simulink model "RemoteMicrogrid"  (R2025a)
settings: Solver=FixedStepAuto  StartTime=0.0  StopTime=8  FixedStep=Ts  MaxStep=1e-3  RelTol=1e-3
PreLoadFcn:
  | RemoteMicrogridInputData
undefined symbols (not defined in the file): BESS, ControlRoom, DiscIntNeverNeededParam, Grid, Load, Machine, Microgrid, MicrogridStatus, PV, relay1, T_on, Ts
libraries: ee_lib x53, fl_lib x39, eeGeneralControl x30, simulink x30, nesl_utility x26, nesl_utility_internal x19, slpidlib x7, eeTransforms x5, eeRmsMeasurement x4, eeTotalHarmonicDistorsion x4, batteryecm_lib x2, simulink_extras x2
(part 4 of 6)

== system RemoteMicrogrid/Diesel Substation, BESS, & Microgrid Controller/Diesel Generator/AVR and Exciter ==
  Constant{3,5..9} (6 alike) : Constant  Value=0
  Constant4 : Constant  Value=1.05
  "E_FD Simulink-PS " : nesl_utility/Simulink-PS Converter  PhysicalDomain=network_engine_domain  SubClassName=ps_input  LeftPortType=input  RightPortType=output  PseudoPeriodic=off  Frequencies=[]  NoiseDistribution=none  NoiseParameters=[]  Unit=1  AffineConversion=off  FilteringAndDerivatives=provide  SimscapeFilterOrder=1  InputFilterTimeConstant=.001  UdotUserProvided=0
  I_FD PS-Simulink : nesl_utility/PS-Simulink Converter  PhysicalDomain=network_engine_domain  SubClassName=ps_output  LeftPortType=input  RightPortType=output  PseudoPeriodic=off  Frequencies=[]  VectorFormat=1-D array  Unit=1  AffineConversion=off
  SM DC2C : eeSmDC2C/SM DC2C  E_FD0=2.5  Ts=Ts  R_C=0  X_C=0  T_R=0  K_A=300  T_A=0.06  T_B=0  T_C=0  K_F=0.058  T_F=0.62  V_Rmax=4.5  V_Rmin=-4.5  oelInputLocation=Unused  uelInputLocation=Unused  sclInputLocation=Unused  K_E=1  T_E=1.33  E_FDmin=-99  E_1=3.05  S_E_E1=0.279  E_2=2.29  S_E_E2=0.117
  Synchronous Machine Field Circuit (pu) : ee_lib/Electromechanical/Synchronous/Synchronous Machine Field Circuit  unit_option=ee.enum.unit.pu  SRated=Grid.DieselRatedPower V*A  FRated=Grid.Frequency Hz  fieldCircuitParameterization_option=ee.enum.sm.fieldparameterization.current  baseEfd=200 V  baseIfd=1300 A  parameterization_option=2  Ladu=1.66  Rfd=0.0006  Xl=0.05  Xd=1.72  Xdd=0.13  Xddd=0.09  d_option=ee.enum.circuit.open  Td0d=0.75 s  Tdd=0.03 s  Td0dd=0.003 s  Tddd=0.008 s
      settings: InternalSimscapePortConfiguration="{\"Bottom\":[],\"Left\":[{\"id\":\"Efd_pu\",\"label\":\"Efd_pu\",\"type\":\"input\"},{\"id\":\"Ifd_pu\",\"label\":\"Ifd_pu\",\"type\":\"output\"}],\"Right\":[{\"id\":\"fd_p\",\"label\":\"fd+\",\"type\":\"foundation.electrical.electrical\"},{\"id\":\"fd_n\",\"label\":\"fd-\",\"type\":\"foundation.electrical.electrical\"}],\"Top\":[]}"
  Terminal Current Measurement : ee_lib/Electromechanical/Synchronous/Synchronous Machine Measurement  output_idx=15
      settings: InternalSimscapePortConfiguration="{\"Bottom\":[],\"Left\":[{\"id\":\"pu_input\",\"label\":\"pu\",\"type\":\"input\"}],\"Right\":[{\"id\":\"pu_output\",\"label\":\"o\",\"type\":\"output\"}],\"Top\":[]}"
  Terminal Current PS-Simulink : nesl_utility/PS-Simulink Converter  PhysicalDomain=network_engine_domain  SubClassName=ps_output  LeftPortType=input  RightPortType=output  PseudoPeriodic=off  Frequencies=[]  VectorFormat=1-D array  Unit=1  AffineConversion=off
  Terminal Voltage Measurement : ee_lib/Electromechanical/Synchronous/Synchronous Machine Measurement  output_idx=14
      settings: InternalSimscapePortConfiguration="{\"Bottom\":[],\"Left\":[{\"id\":\"pu_input\",\"label\":\"pu\",\"type\":\"input\"}],\"Right\":[{\"id\":\"pu_output\",\"label\":\"o\",\"type\":\"output\"}],\"Top\":[]}"
  Terminal Voltage PS-Simulink : nesl_utility/PS-Simulink Converter  PhysicalDomain=network_engine_domain  SubClassName=ps_output  LeftPortType=input  RightPortType=output  PseudoPeriodic=off  Frequencies=[]  VectorFormat=1-D array  Unit=1  AffineConversion=off
  Terminator : Terminator
  pu : PMIOPort  Side=Left
  fd+ : PMIOPort  Port=2  Side=Right
  fd- : PMIOPort  Port=3  Side=Right
  wires:
  Terminal Current PS-Simulink/1 -> SM DC2C/4
  SM DC2C/1 -> "E_FD Simulink-PS "/1
  Constant9/1 -> SM DC2C/9
  Constant8/1 -> SM DC2C/8
  Constant7/1 -> SM DC2C/7
  Constant6/1 -> SM DC2C/6
  Constant5/1 -> SM DC2C/5
  Constant3/1 -> SM DC2C/2
  I_FD PS-Simulink/1 -> Terminator/1
  Constant4/1 -> SM DC2C/1
  Terminal Voltage PS-Simulink/1 -> SM DC2C/3
  connections:
  Terminal Current Measurement/RConn1 -- Terminal Current PS-Simulink/LConn1
  Terminal Voltage Measurement/RConn1 -- Terminal Voltage PS-Simulink/LConn1
  pu/RConn1 -- Terminal Current Measurement/LConn1 -- Terminal Voltage Measurement/LConn1
  Synchronous Machine Field Circuit (pu)/RConn1 -- fd+/RConn1
  fd-/RConn1 -- Synchronous Machine Field Circuit (pu)/RConn2
  I_FD PS-Simulink/LConn1 -- Synchronous Machine Field Circuit (pu)/LConn2
  "E_FD Simulink-PS "/RConn1 -- Synchronous Machine Field Circuit (pu)/LConn1

== system RemoteMicrogrid/Diesel Substation, BESS, & Microgrid Controller/Diesel Generator/Governor and Prime Mover  ==
  Load : Inport
  Governor : Subsystem
  Ideal Torque Source : fl_lib/Mechanical/Mechanical Sources/Ideal Torque Source
  Mechanical Rotational Reference : fl_lib/Mechanical/Rotational Elements/Mechanical Rotational Reference
  Non-reheat turbine : Subsystem
  PS-Simulink Converter : nesl_utility/PS-Simulink Converter  PhysicalDomain=network_engine_domain  SubClassName=ps_output  LeftPortType=input  RightPortType=output  PseudoPeriodic=off  Frequencies=[]  VectorFormat=1-D array  Unit=1  AffineConversion=off
  Rotor Velocity Measurement : ee_lib/Electromechanical/Synchronous/Synchronous Machine Measurement  output_idx=4
      settings: InternalSimscapePortConfiguration="{\"Bottom\":[],\"Left\":[{\"id\":\"pu_input\",\"label\":\"pu\",\"type\":\"input\"}],\"Right\":[{\"id\":\"pu_output\",\"label\":\"o\",\"type\":\"output\"}],\"Top\":[]}"
  Simulink-PS Converter : nesl_utility/Simulink-PS Converter  PhysicalDomain=network_engine_domain  SubClassName=ps_input  LeftPortType=input  RightPortType=output  PseudoPeriodic=off  Frequencies=[]  NoiseDistribution=none  NoiseParameters=[]  Unit=1  AffineConversion=off  FilteringAndDerivatives=zero  SimscapeFilterOrder=1  InputFilterTimeConstant=0.001  UdotUserProvided=1
  scale by base_torque : Gain  Gain=base_torque
  R : PMIOPort  Side=Right
  C : PMIOPort  Port=2  Side=Right
  pu : PMIOPort  Port=3  Side=Left
  wires:
  PS-Simulink Converter/1 -> Governor/1(pu_velocity)
  Governor/1(delta_y) -> Non-reheat turbine/1(delta_y)
  Non-reheat turbine/1(torque) -> scale by base_torque/1
  scale by base_torque/1 -> Simulink-PS Converter/1
  Load/1 -> Governor/2(Load Reference)
  connections:
  C/RConn1 -- Ideal Torque Source/RConn2 -- Mechanical Rotational Reference/LConn1
  Ideal Torque Source/LConn1 -- R/RConn1
  pu/RConn1 -- Rotor Velocity Measurement/LConn1
  PS-Simulink Converter/LConn1 -- Rotor Velocity Measurement/RConn1
  Simulink-PS Converter/RConn1 -- Ideal Torque Source/RConn1

== system RemoteMicrogrid/Diesel Substation, BESS, & Microgrid Controller/Microgrid Controller/Breaker Control ==
  Bus Element In : Inport  PortName=BrKControl  Element=PCC
  CtrlRm BRK : Inport  Port=2
  Cast To Double1 : DataTypeConversion  OutDataTypeStr=double  SaturateOnIntegerOverflow=off  RndMeth=Floor
  Delay : Delay  DelayLength=1  InitialCondition=ControlRoom.BRKInitialStatus
  Switch : Switch  Criteria=u2 > Threshold  SaturateOnIntegerOverflow=off  InputSameDT=off
  BrK Ctrl : Outport
  wires:
  Delay/1 -> Cast To Double1/1
  Bus Element In/1 -> Delay/1
  CtrlRm BRK/1 -> Switch/1, Switch/2
  Cast To Double1/1 -> Switch/3  "BRK Status"
  Switch/1 -> BrK Ctrl/1  "BRK Status"

== system RemoteMicrogrid/Diesel Substation, BESS, & Microgrid Controller/Microgrid Controller/Microgrid Control Functions ==
  PLL : Inport
  BESS Reactive Power : Inport  Port=2
  PCC Active Power : Inport  Port=3
  PCC Reactive Power : Inport  Port=4
  Bus Element In1 : Inport  Port=5  PortName=Status  Element=plannedIslandingEnable
  Bus Element In2 : Inport  Port=5  PortName=Status  Element=blackStart
  Bus Element In4 : Inport  Port=5  PortName=Status  Element=resyncEnable
  Bus Element In3 : Inport  Port=5  PortName=Status  Element=resync
  Data Type Conversion : DataTypeConversion  OutDataTypeStr=boolean  SaturateOnIntegerOverflow=off  RndMeth=Floor
  Latency_PlannedIsland : Delay  DelayLength=1  SampleTime=Ts
  Latency_Resync : Delay  DelayLength=1  SampleTime=Ts
  Model : ModelReference  ModelNameDialog=Resynchronization.slx  UsingDefaultArgumentValue=0,0,0,0,0,0,0,0,0,0,0  SimulationMode=Normal  ModelReferenceVersion=5.0  GridFrequency=gridFrequency  KpVolResynch=kpVoltage  KiVolResynch=kiVoltage  VoltageThreshold=voltageThreshold  kDroop=voltageDroop  KpFreResynch=kpFrequency  KiFreResynch=kiFrequency  FrequencyThreshold=frequencyThreshold  KpAngResynch=kpAngle  KiAngResynch=kiAngle  AngleThreshold=angleThreshold
  Model1 : ModelReference  ModelNameDialog=PlannedIsland.slx  UsingDefaultArgumentValue=0,0,0,0,0,0  SimulationMode=Normal  ModelReferenceVersion=5.0  KpPPlannedIsland=kpActive  KiPPlannedIsland=kiActive  ZeroActivePowerThreshold=activeThreshold  KpQPlannedIsland=kpReactive  KiQPlannedIsland=kiReactive  ZeroReactivePowerThreshold=reactiveThreshold
  Model2 : ModelReference  ModelNameDialog=Black_Start.slx  UsingDefaultArgumentValue=0,0,0,0,0,0,0,0  SimulationMode=Normal  ModelReferenceVersion=5.0  referenceFrequency=gridFrequency  controllerBlackStart=blackStartTime  voltageLevel1=level1  voltageLevel2=level2  voltageLevel3=level3  delayLevel1=delay1  delayLevel2=delay2  delayLevel3=delay3
  Terminator : Terminator
  Resync : Outport
  PlannedIslanding : Outport  Port=2
  BlackStart : Outport  Port=3
  Resync Status : Outport  Port=4
  PlannedIsland Status : Outport  Port=5
  wires:
  Model1/2 -> PlannedIslanding/1  "PlannedIslanding"
  PCC Reactive Power/1 -> Model1/3
  PCC Active Power/1 -> Model1/2
  Model/1 -> Latency_Resync/1
  Model1/1 -> Latency_PlannedIsland/1
  Bus Element In2/1 -> Model2/1
  Model2/1 -> BlackStart/1  "BlackStart"
  Bus Element In1/1 -> Model1/1
  Model/2 -> Resync/1  "Resync"
  Bus Element In3/1 -> Data Type Conversion/1
  Bus Element In4/1 -> Model/1
  BESS Reactive Power/1 -> Model/2
  PLL/1 -> Model2/2, Model/3
  Data Type Conversion/1 -> Model/4
  Latency_Resync/1 -> Resync Status/1
  Latency_PlannedIsland/1 -> PlannedIsland Status/1
  Model2/2 -> Terminator/1

== system RemoteMicrogrid/Diesel Substation, BESS, & Microgrid Controller/Microgrid Controller/Microgrid Supervisory Control ==
  Resync Status : Inport
  PlannedIslanding Status : Inport  Port=2
  Resync Enable : Inport  Port=3
  PlannedIslandEnable : Inport  Port=4
  UnplannedIslandingEnable : Inport  Port=5
  Bus Element In : Inport  Port=6  PortName=mPLL  Element=Island.voltage
  Bus Element In1 : Inport  Port=6  PortName=mPLL  Element=Island.frequency
  BreakerStatus : Inport  Port=7
  Bus Assignment : BusAssignment  AssignedSignals=mode
  Bus Creator : BusCreator  Inputs=3
  Bus Creator1 : BusCreator  Inputs=2
  Bus Creator2 : BusCreator  Inputs=3
  Constant : Constant  Value=resyncDelay
  Constant1 : Constant  Value=plannedIslandingDelay
  Delay : Delay  DelayLength=1  InitialCondition=ControlRoom.BRKInitialStatus  SampleTime=Ts
  Scope : Scope
      settings: ActiveDisplayYMinimum=0.75  ActiveDisplayYMaximum=3.25
  Transition and Dispatch Control : Stateflow chart  TreatAsAtomicUnit=on  mask(Microgrid Transition and Dispatch Control){upperVoltageLimit=upperVoltagelimit, lowerVoltageLimit=lowerVoltageLimit, upperFrequencyLimit=upperFrequencyLimit, lowerFrequencyLimit=lowerFrequencyLimit}
      mask prompts: upperVoltageLimit "Max Voltage in pu"; lowerVoltageLimit "Min Voltage in pu"; upperFrequencyLimit "Max Frequency in Hz"; lowerFrequencyLimit "Min Frequency in Hz"
      mask help: This subsystem implements the transitions and the corresponding dispatch functions in the microgrid
  BrKControl : Outport
  Status : Outport  Port=2
  wires:
  Constant1/1 -> Bus Creator2/3  "delay"
  PlannedIslanding Status/1 -> Bus Creator2/2  "status"
  PlannedIslandEnable/1 -> Bus Creator2/1  "enable"
  Bus Creator2/1 -> Transition and Dispatch Control/5(PlannedIslanding)  "PlannedIslanding"
  UnplannedIslandingEnable/1 -> Transition and Dispatch Control/2(UnplannedIslandingEnable)
  Bus Creator1/1 -> Transition and Dispatch Control/3(Island)  "Island"
  Bus Element In1/1 -> Bus Creator1/2  "frequency"
  Bus Element In/1 -> Bus Creator1/1  "voltage"
  Bus Creator/1 -> Transition and Dispatch Control/1(Resync)  "Resync"
  Constant/1 -> Bus Creator/3  "delay"
  Resync Status/1 -> Bus Creator/2  "status"
  Resync Enable/1 -> Bus Creator/1  "enable"
  Transition and Dispatch Control/1(BrKControl) -> BrKControl/1  "BrKControl"
  BreakerStatus/1 -> Delay/1
  Delay/1 -> Transition and Dispatch Control/4(BreakerStatus)
  Transition and Dispatch Control/2(Status) -> Bus Assignment/1
  Transition and Dispatch Control/3(Transition_and_Dispatch_ControlMode) -> Bus Assignment/2, Scope/1
  Bus Assignment/1 -> Status/1  "Status"

== system RemoteMicrogrid/Diesel Substation, BESS, & Microgrid Controller/PCC Measurements and PCC Breaker/Circuit Breaker ==
  BRK : Inport
  Data Type Conversion : DataTypeConversion  OutDataTypeStr=double  SaturateOnIntegerOverflow=off  RndMeth=Floor
  Open Resistance : Gain  Gain=1e5
  Phase Splitter : ee_lib/Connectors & References/Phase Splitter
  Phase Splitter1 : ee_lib/Connectors & References/Phase Splitter
  Simulink-PS Converter : nesl_utility/Simulink-PS Converter  PhysicalDomain=network_engine_domain  SubClassName=ps_input  LeftPortType=input  RightPortType=output  PseudoPeriodic=off  Frequencies=[]  NoiseDistribution=none  NoiseParameters=[]  Unit=1  AffineConversion=off  FilteringAndDerivatives=provide  SimscapeFilterOrder=1  InputFilterTimeConstant=0.001  UdotUserProvided=0
  Variable Resistor : fl_lib/Electrical/Electrical Elements/Variable Resistor  Rmin=1e-3 Ohm  thermalEnable=false  thermal_mass=1 J/K  i_specify=off  i_priority=None  i=0 A  i_nominal_specify=off  i_nominal_value=1  i_nominal_unit=A  v_specify=off  v_priority=None  v=0 V  v_nominal_specify=off  v_nominal_value=1  v_nominal_unit=V  T_specify=off  T_priority=None  T=300 K  T_nominal_specify=off  T_nominal_value=1  T_nominal_unit=K
  Variable Resistor1 : fl_lib/Electrical/Electrical Elements/Variable Resistor  Rmin=1e-3 Ohm  thermalEnable=false  thermal_mass=1 J/K  i_specify=off  i_priority=None  i=0 A  i_nominal_specify=off  i_nominal_value=1  i_nominal_unit=A  v_specify=off  v_priority=None  v=0 V  v_nominal_specify=off  v_nominal_value=1  v_nominal_unit=V  T_specify=off  T_priority=None  T=300 K  T_nominal_specify=off  T_nominal_value=1  T_nominal_unit=K
  Variable Resistor2 : fl_lib/Electrical/Electrical Elements/Variable Resistor  Rmin=1e-3 Ohm  thermalEnable=false  thermal_mass=1 J/K  i_specify=off  i_priority=None  i=0 A  i_nominal_specify=off  i_nominal_value=1  i_nominal_unit=A  v_specify=off  v_priority=None  v=0 V  v_nominal_specify=off  v_nominal_value=1  v_nominal_unit=V  T_specify=off  T_priority=None  T=300 K  T_nominal_specify=off  T_nominal_value=1  T_nominal_unit=K
  In : PMIOPort  Side=Left
  ~ : PMIOPort  Port=2  Side=Right
  wires:
  Data Type Conversion/1 -> Open Resistance/1
  BRK/1 -> Data Type Conversion/1
  Open Resistance/1 -> Simulink-PS Converter/1
  connections:
  Phase Splitter1/RConn2 -- Variable Resistor1/RConn1
  Variable Resistor1/LConn2 -- Phase Splitter/RConn2
  Phase Splitter1/RConn3 -- Variable Resistor2/RConn1
  Phase Splitter/RConn1 -- Variable Resistor/LConn2
  Variable Resistor2/LConn2 -- Phase Splitter/RConn3
  Phase Splitter1/RConn1 -- Variable Resistor/RConn1
  Phase Splitter1/LConn1 -- ~/RConn1
  Variable Resistor/LConn1 -- Simulink-PS Converter/RConn1 -- Variable Resistor2/LConn1 -- Variable Resistor1/LConn1
  Phase Splitter/LConn1 -- In/RConn1

== system RemoteMicrogrid/Diesel Substation, BESS, & Microgrid Controller/PCC Measurements and PCC Breaker/Diesel Genset Current Measurement ==
  Current and Voltage Sensor (Three-Phase)1 : ee_lib/Sensors & Transducers/Current and Voltage Sensor (Three-Phase)  vMeasurementType=ee.enum.vmeasurement.ll  outputUnit=ee.enum.unit.pu  SRated=150e3 A*V  VRated=Microgrid.Voltage V  I_specify=off  I_priority=None  I=[0, 0, 0] A  I_nominal_specify=off  I_nominal_value=1  I_nominal_unit=A  V_specify=off  V_priority=None  V=[0, 0, 0] V  V_nominal_specify=off  V_nominal_value=1  V_nominal_unit=V
      settings: InternalSimscapePortConfiguration="{\"Bottom\":[],\"Left\":[{\"id\":\"N1\",\"label\":\"~1\",\"type\":\"foundation.electrical.three_phase\"}],\"Right\":[{\"id\":\"V_output\",\"label\":\"V\",\"type\":\"output\"},{\"id\":\"I_output\",\"label\":\"I\",\"type\":\"output\"},{\"id\":\"N2\",\"label\":\"~2\",\"type\":\"foundation.electrical.three_phase\"}],\"Top\":[]}"
  PS-Simulink Converter2 : nesl_utility_internal/PS-Simulink Converter  PhysicalDomain=network_engine_domain  SubClassName=ps_output  LeftPortType=input  RightPortType=output  PseudoPeriodic=off  Frequencies=[]  VectorFormat=1-D array  Unit=V  AffineConversion=off
  PS-Simulink Converter3 : nesl_utility_internal/PS-Simulink Converter  PhysicalDomain=network_engine_domain  SubClassName=ps_output  LeftPortType=input  RightPortType=output  PseudoPeriodic=off  Frequencies=[]  VectorFormat=1-D array  Unit=A  AffineConversion=off
  Terminator : Terminator
  ~ : PMIOPort  Side=Left
  "~ " : PMIOPort  Port=2  Side=Right
  Out Bus Element : Outport  PortName=Grid  Element=voltage
  wires:
  PS-Simulink Converter3/1 -> Terminator/1
  PS-Simulink Converter2/1 -> Out Bus Element/1
  connections:
  Current and Voltage Sensor (Three-Phase)1/RConn1 -- PS-Simulink Converter2/LConn1
  ~/RConn1 -- Current and Voltage Sensor (Three-Phase)1/LConn1
  Current and Voltage Sensor (Three-Phase)1/RConn2 -- PS-Simulink Converter3/LConn1
  Current and Voltage Sensor (Three-Phase)1/RConn3 -- "~ "/RConn1

== system RemoteMicrogrid/Diesel Substation, BESS, & Microgrid Controller/PCC Measurements and PCC Breaker/Diesel Genset Power Measurement ==
  Current and Voltage Sensor (Three-Phase) : ee_lib/Sensors & Transducers/Current and Voltage Sensor (Three-Phase)  vMeasurementType=ee.enum.vmeasurement.ll  outputUnit=ee.enum.unit.pu  SRated=150e3 A*V  VRated=Microgrid.Voltage V  I_specify=off  I_priority=None  I=[0, 0, 0] A  I_nominal_specify=off  I_nominal_value=1  I_nominal_unit=A  V_specify=off  V_priority=None  V=[0, 0, 0] V  V_nominal_specify=off  V_nominal_value=1  V_nominal_unit=V
      settings: InternalSimscapePortConfiguration="{\"Bottom\":[],\"Left\":[{\"id\":\"N1\",\"label\":\"~1\",\"type\":\"foundation.electrical.three_phase\"}],\"Right\":[{\"id\":\"V_output\",\"label\":\"V\",\"type\":\"output\"},{\"id\":\"I_output\",\"label\":\"I\",\"type\":\"output\"},{\"id\":\"N2\",\"label\":\"~2\",\"type\":\"foundation.electrical.three_phase\"}],\"Top\":[]}"
  Low-Pass Filter (Discrete or Continuous) : eeGeneralControl/Low-Pass Filter (Discrete or Continuous)  K=1  T=0.02  B=inf  A=-inf  init_option=Inherited from block input  x0=0  Ts=Ts
  Low-Pass Filter (Discrete or Continuous)1 : eeGeneralControl/Low-Pass Filter (Discrete or Continuous)  K=1  T=0.02  B=inf  A=-inf  init_option=Inherited from block input  x0=0  Ts=Ts
  PS-Simulink Converter : nesl_utility_internal/PS-Simulink Converter  PhysicalDomain=network_engine_domain  SubClassName=ps_output  LeftPortType=input  RightPortType=output  PseudoPeriodic=off  Frequencies=[]  VectorFormat=1-D array  Unit=inherit  AffineConversion=off
  PS-Simulink Converter1 : nesl_utility_internal/PS-Simulink Converter  PhysicalDomain=network_engine_domain  SubClassName=ps_output  LeftPortType=input  RightPortType=output  PseudoPeriodic=off  Frequencies=[]  VectorFormat=1-D array  Unit=inherit  AffineConversion=off
  PS-Simulink Converter8 : nesl_utility_internal/PS-Simulink Converter  PhysicalDomain=network_engine_domain  SubClassName=ps_output  LeftPortType=input  RightPortType=output  PseudoPeriodic=off  Frequencies=[]  VectorFormat=1-D array  Unit=kW  AffineConversion=off
  PS-Simulink Converter9 : nesl_utility_internal/PS-Simulink Converter  PhysicalDomain=network_engine_domain  SubClassName=ps_output  LeftPortType=input  RightPortType=output  PseudoPeriodic=off  Frequencies=[]  VectorFormat=1-D array  Unit=kV*A  AffineConversion=off
  Power Sensor (Three-Phase)2 : ee_lib/Sensors & Transducers/Power Sensor (Three-Phase)  load_type=ee.enum.passive.type_balanced.balanced  f0=60 Hz  config=ee.enum.with_neutral.no  rho=1
      settings: InternalSimscapePortConfiguration="{\"Bottom\":[],\"Left\":[{\"id\":\"N1\",\"label\":\"~1\",\"type\":\"foundation.electrical.three_phase\"}],\"Right\":[{\"id\":\"N2\",\"label\":\"~2\",\"type\":\"foundation.electrical.three_phase\"}],\"Top\":[{\"id\":\"Pm\",\"label\":\"P\",\"type\":\"output\"},{\"id\":\"Qm\",\"label\":\"Q\",\"type\":\"output\"}]}"
  ~ : PMIOPort  Side=Left
  "~ " : PMIOPort  Port=2  Side=Right
  Out Bus Element : Outport  PortName=PCC  Element=voltage
  Out Bus Element1 : Outport  PortName=PCC  Element=current
  Out Bus Element2 : Outport  PortName=PCC  Element=activePower
  Out Bus Element3 : Outport  PortName=PCC  Element=reactivePower
  wires:
  PS-Simulink Converter8/1 -> Low-Pass Filter (Discrete or Continuous)/1
  PS-Simulink Converter9/1 -> Low-Pass Filter (Discrete or Continuous)1/1
  PS-Simulink Converter1/1 -> Out Bus Element1/1
  Low-Pass Filter (Discrete or Continuous)/1 -> Out Bus Element2/1
  Low-Pass Filter (Discrete or Continuous)1/1 -> Out Bus Element3/1
  PS-Simulink Converter/1 -> Out Bus Element/1
  connections:
  Current and Voltage Sensor (Three-Phase)/RConn2 -- PS-Simulink Converter1/LConn1
  PS-Simulink Converter/LConn1 -- Current and Voltage Sensor (Three-Phase)/RConn1
  Power Sensor (Three-Phase)2/RConn1 -- Current and Voltage Sensor (Three-Phase)/LConn1
  PS-Simulink Converter9/LConn1 -- Power Sensor (Three-Phase)2/LConn3
  Current and Voltage Sensor (Three-Phase)/RConn3 -- "~ "/RConn1
  PS-Simulink Converter8/LConn1 -- Power Sensor (Three-Phase)2/LConn2
  ~/RConn1 -- Power Sensor (Three-Phase)2/LConn1

== system RemoteMicrogrid/Operator Control Room/Measurements and Visualizations /Mode Selection ==
  Mode : Inport
  Mode-0 : simulink/Logic and Bit Operations/Compare To Constant  relop===  const=MicrogridStatus.None  OutDataTypeStr=boolean
  Mode-1 : simulink/Logic and Bit Operations/Compare To Constant  relop===  const=MicrogridStatus.Steady_State_Islanded  OutDataTypeStr=boolean
  Mode-2 : simulink/Logic and Bit Operations/Compare To Constant  relop===  const=MicrogridStatus.Resynchronization  OutDataTypeStr=boolean
  Mode-3 : simulink/Logic and Bit Operations/Compare To Constant  relop===  const=MicrogridStatus.Steady_State_Grid_Connected  OutDataTypeStr=boolean
  Mode-4 : simulink/Logic and Bit Operations/Compare To Constant  relop===  const=MicrogridStatus.Planned_Islanding  OutDataTypeStr=boolean
  Mode-5 : simulink/Logic and Bit Operations/Compare To Constant  relop===  const=MicrogridStatus.Unplanned_Islanding  OutDataTypeStr=boolean
  Scope : Scope  NumInputPorts=6
      settings: ActiveDisplayYMinimum=-0.125  ActiveDisplayYMaximum=1.125  DataLoggingVariableName=ScopeData3
  wires:
  Mode/1 -> Mode-2/1, Mode-0/1, Mode-1/1, Mode-3/1, Mode-5/1, Mode-4/1
  Mode-0/1 -> Scope/1  "Mode-0"
  Mode-1/1 -> Scope/2  "Mode-1"
  Mode-2/1 -> Scope/3  "Mode-2"
  Mode-3/1 -> Scope/4  "Mode-3"
  Mode-4/1 -> Scope/5  "Mode-4"
  Mode-5/1 -> Scope/6  "Mode-5"

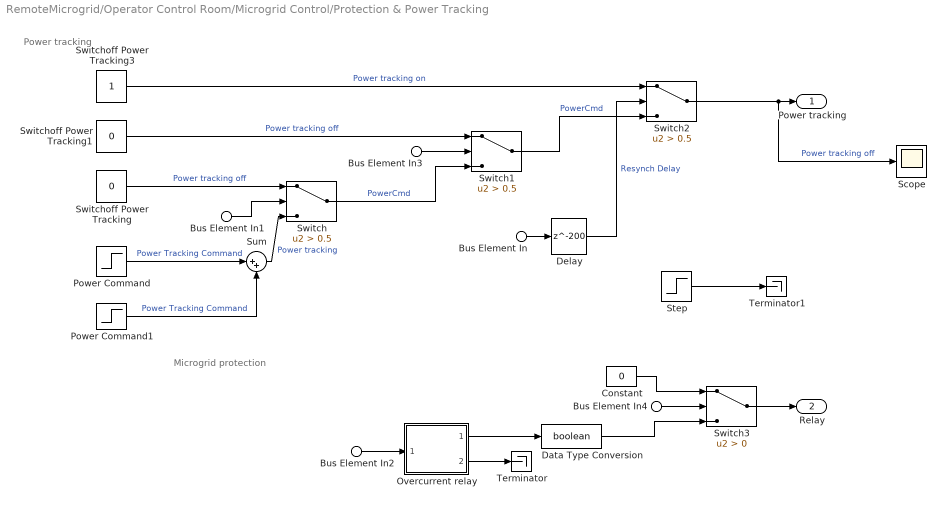
== system RemoteMicrogrid/Operator Control Room/Microgrid Control/Protection & Power Tracking ==
  note: Power tracking
  note: Microgrid protection
  Bus Element In1 : Inport  PortName=MGSubstation  Element=MGController.BRK Status
  Bus Element In4 : Inport  PortName=MGSubstation  Element=MGController.BRK Status
  Bus Element In : Inport  PortName=MGSubstation  Element=MGController.Status.resyncEnable
  Bus Element In3 : Inport  PortName=MGSubstation  Element=MGController.Status.resync
  Bus Element In2 : Inport  PortName=MGSubstation  Element=mPCC.PCC.current
  Constant : Constant  Value=0  OutDataTypeStr=boolean
  Data Type Conversion : DataTypeConversion  OutDataTypeStr=boolean  SaturateOnIntegerOverflow=off  RndMeth=Floor
  Delay : Delay  DelayLength=200  SampleTime=1000*Ts
  Overcurrent relay : Subsystem  SystemSampleTime=relay1.sampleTime  mask{relayCharacteristicPhase=Definite Time, relayCharacteristicEarth=Definite Time, ratedFrequency=60, sampleTime=Ts, protectionEnable=1, currentPhase=[1.5 2.5 3.5 4.5 5.5 6.5 7.5 8.5 9.5 10.5], tmsPhase=[0.1 0.2], topPhase=[0.64 1.29;0.29 0.58;0.21 0.43;0.18 0.36;0.16 0.32;0.15 0.29;0.14 0.27;0.13 0.26;0.12 0.25;0.12 0.24], currentEarth=[0.06 0.15 0.2 0.25 0.3 0.35 0.4 0.45 0.5 0.55], tmsEarth=[0.1 0.2], topEarth=[0.64 1.29;0.29 0.58;0.21 0.43;0.18 0.36;0.16 0.32;0.15 0.29;0.14 0.27;0.13 0.26;0.12 0.25;0.12 0.24], phPickUp=1.1, ethPickUp=0.01, phTimeSetting=0.1, ethTimeSetting=0.1, topPhaseActual=0.5, topEarthActual=0.3}
      mask prompts: relayCharacteristicPhase "Relay characteristics for phase protection"; relayCharacteristicEarth "Relay characteristics for earth protection"; ratedFrequency "Fundamental frequency (Hz)"; sampleTime "Relay sample time (s)"; protectionEnable "Relay operation enable"; currentPhase "Current setting for phase protection (A)"; tmsPhase "Time multiplier setting for phase protection (s)"; topPhase "Operating time for phase protection (s)"; currentEarth "Current setting for earth protection (A)"; tmsEarth "Time multiplier setting for earth protection (s)"; topEarth "Operating time for earth protection (s)"; phPickUp "Pick up current for phase protection (A)"; ethPickUp "Pick up current for earth protection (A)"; phTimeSetting "Time multiplier setting for phase protection (s)"; ethTimeSetting "Time multiplier setting for earth protection (s)"; topPhaseActual "Relay operating time for phase protection (s)"; topEarthActual "Relay operating time for earth protection (s)"
      mask TypeOptions relayCharacteristicPhase: IEC Normal Inverse | IEC Very Inverse | IEC Extremely Inverse | IEEE Moderately Inverse | IEEE Very Inverse | IEEE Extremely Inverse | Definite Time | IvsT
      mask Callback relayCharacteristicPhase:
      | % Control parameter visiblity
      | enablePhase = get_param(gcb,'relayCharacteristicPhase');
      | enableEarth = get_param(gcb,'relayCharacteristicEarth');
      | % Set the 'MaskVisibilities' property for each parameters
      | cArray=cell(1,17);
      | cArray(:)={'on'};
      | p=strcmp(enablePhase,'IvsT');
      | q=strcmp(enableEarth,'IvsT');
      | r=strcmp(enablePhase,'Definite Time');
      | s=strcmp(enableEarth,'Definite Time');
      | if p==0 && q==1
      |     cArray(6:8)={'off'};
      | elseif p==0 && q==0
      |     cArray(6:11)={'off'};
      | elseif p==1 && q==0
      |     cArray(9:11)={'off'};
      | end
      | if r==0 && s==1
      |     cArray(15)={'off'};
      |     cArray(16)={'off'};
      | elseif r==0 && s==0
      |     cArray(16:17)={'off'};
      | elseif r==1 && s==0
      |     cArray(14)={'off'};
      |     cArray(17)={'off'};
      | elseif r==1 && s==1
      |     cArray(14:15)={'off'};
      | end
      | set_param(gcb,'MaskVisibilities',cArray);
      mask TypeOptions relayCharacteristicEarth: IEC Normal Inverse | IEC Very Inverse | IEC Extremely Inverse | IEEE Moderately Inverse | IEEE Very Inverse | IEEE Extremely Inverse | Definite Time | IvsT
      mask Callback relayCharacteristicEarth:
      | % Control parameter visiblity
      | enablePhase = get_param(gcb,'relayCharacteristicPhase');
      | enableEarth = get_param(gcb,'relayCharacteristicEarth');
      | % Set the 'MaskVisibilities' property for each parameters
      | cArray=cell(1,17);
      | cArray(:)={'on'};
      | p=strcmp(enablePhase,'IvsT');
      | q=strcmp(enableEarth,'IvsT');
      | r=strcmp(enablePhase,'Definite Time');
      | s=strcmp(enableEarth,'Definite Time');
      | if p==0 && q==1
      |     cArray(6:8)={'off'};
      | elseif p==0 && q==0
      |     cArray(6:11)={'off'};
      | elseif p==1 && q==0
      |     cArray(9:11)={'off'};
      | end
      | if r==0 && s==1
      |     cArray(15)={'off'};
      |     cArray(16)={'off'};
      | elseif r==0 && s==0
      |     cArray(16:17)={'off'};
      | elseif r==1 && s==0
      |     cArray(14)={'off'};
      |     cArray(17)={'off'};
      | elseif r==1 && s==1
      |     cArray(14:15)={'off'};
      | end
      | set_param(gcb,'MaskVisibilities',cArray);
      mask DialogControl Container9 Prompt: Main
      mask DialogControl Container24 Prompt: Current Settings
      mask DialogControl Container19 Prompt: Time Settings
      mask Display:
      | psm = 1:1:30; % Plug setting multiplier
      | tms=0.01; % Time multiplier setting is assumed to be 0.01s
      | top=ones(2,length(psm));  % Operating time of the relay
      | maskParameter=Simulink.Mask.get(gcb); % Get the mask parameters
      | for i=1:2
      |     index(i)=find(strcmp(maskParameter.Parameters(1,i).Value,maskParameter.Parameters(1,i).TypeOptions));
      |     if index(i)<7
      |         switch index(i)              % Selection of relay characteristic
      |             case 1                   % IEC Normal Inverse
      |                 a=0.14;
      |                 b=0.02;
      |                 c=0;
      |             case 2                   % IEC Very Inverse
      |                 a=13.5;
      |                 b=1;
      |                 c=0;
      |             case 3                   % IEC Extremely Inverse
      |                 a=80;
      |                 b=2;
      |                 c=0;
      |             case 4                   % IEEE Moderately Inverse
      |                 a=0.0515;
      |                 b=0.02;
      |                 c=0.114;
      |             case 5                   % IEEE Very Inverse
      |                 a=19.61;
      |                 b=2;
      |                 c=0.491;
      |             otherwise                % IEEE Exteremely Inverse
      |                 a=28.2;
      |                 b=2;
      |                 c=0.1217;
      |         end
      |         for j=1:length(psm)
      |             top(i,j)=tms*((a/(power(psm(j),b)-1))+c); % Operating time of the relay
      |         end
      |     else
      |         top(i,1:length(psm))=0.03*ones(1,length(psm));% Operating time of the relay
      |     end
      | end
      | top1=top(1,1:end);
      | top2=top(2,1:end);
      | 
      | maskFigure=figure;
      | if index(1)<8
      |     plot(psm,top1)
      | else
      |     fprintf('\n\nIvsT');
      | end
      | hold on;
      | if index(2)<8
      |     plot(psm,top2);
      | elseif index(1)<8
      |     fprintf('\nIvsT');
      | end
      | close(maskFigure);
  Power Command : Step  Time=0.5  SampleTime=Ts
  Power Command1 : Step  Time=50  After=-1  SampleTime=Ts
  Scope : Scope
      settings: ActiveDisplayYMinimum=-1  ActiveDisplayYMaximum=1  DataLoggingVariableName=ScopeData3
  Step : Step  Time=ControlRoom.unplannedIslanding  SampleTime=0
  Sum : Sum  Inputs=|++
  Switch : Switch  Criteria=u2 > Threshold  Threshold=0.5  SaturateOnIntegerOverflow=off  InputSameDT=off
  Switch1 : Switch  Criteria=u2 > Threshold  Threshold=0.5  SaturateOnIntegerOverflow=off  InputSameDT=off
  Switch2 : Switch  Criteria=u2 > Threshold  Threshold=0.5  SaturateOnIntegerOverflow=off  InputSameDT=off
  Switch3 : Switch  Criteria=u2 > Threshold  SaturateOnIntegerOverflow=off  InputSameDT=off
  Switchoff Power Tracking : Constant  Value=0
  Switchoff Power Tracking1 : Constant  Value=0
  Switchoff Power Tracking3 : Constant
  Terminator : Terminator
  Terminator1 : Terminator
  Power tracking : Outport
  Relay : Outport  Port=2
  wires:
  Switchoff Power Tracking/1 -> Switch/1  "Power tracking off"
  Bus Element In1/1 -> Switch/2
  Delay/1 -> Switch2/2  "Resynch Delay"
  Sum/1 -> Switch/3  "Power tracking"
  Power Command1/1 -> Sum/2  "Power Tracking Command"
  Power Command/1 -> Sum/1  "Power Tracking Command"
  Switchoff Power Tracking3/1 -> Switch2/1  "Power tracking on"
  Switch/1 -> Switch1/3  "PowerCmd"
  Switch1/1 -> Switch2/3  "PowerCmd"
  Switchoff Power Tracking1/1 -> Switch1/1  "Power tracking off"
  Bus Element In/1 -> Delay/1
  Switch2/1 -> Scope/1, Power tracking/1  "Power tracking off"
  Bus Element In2/1 -> Overcurrent relay/1(Inport)
  Overcurrent relay/1(Trip Signal) -> Data Type Conversion/1
  Bus Element In3/1 -> Switch1/2
  Overcurrent relay/2(Relay Status) -> Terminator/1
  Step/1 -> Terminator1/1
  Data Type Conversion/1 -> Switch3/3
  Bus Element In4/1 -> Switch3/2
  Switch3/1 -> Relay/1
  Constant/1 -> Switch3/1

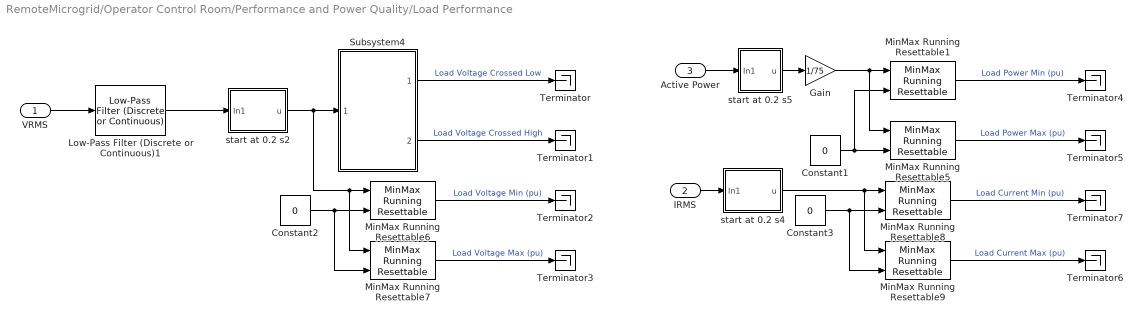
== system RemoteMicrogrid/Operator Control Room/Performance and Power Quality/Load Performance  ==
  VRMS : Inport
  IRMS : Inport  Port=2
  Active Power : Inport  Port=3
  Constant1 : Constant  Value=0
  Constant2 : Constant  Value=0
  Constant3 : Constant  Value=0
  Gain : Gain  Gain=1/75
  Low-Pass Filter (Discrete or Continuous)1 : eeGeneralControl/Low-Pass Filter (Discrete or Continuous)  K=1  T=0.04  B=inf  A=-inf  init_option=Inherited from block input  x0=0  Ts=Ts
  MinMax Running Resettable1 : simulink/Math Operations/MinMax Running Resettable  Function=min  vinit=1
  MinMax Running Resettable5 : simulink/Math Operations/MinMax Running Resettable  Function=max  vinit=1
  MinMax Running Resettable6 : simulink/Math Operations/MinMax Running Resettable  Function=min  vinit=1
  MinMax Running Resettable7 : simulink/Math Operations/MinMax Running Resettable  Function=max  vinit=1
  MinMax Running Resettable8 : simulink/Math Operations/MinMax Running Resettable  Function=min  vinit=0.707
  MinMax Running Resettable9 : simulink/Math Operations/MinMax Running Resettable  Function=max  vinit=0.491
  Subsystem4 : Subsystem
  Terminator{,1..7} (8 alike) : Terminator
  start at 0.2 s2 : Subsystem
  start at 0.2 s4 : Subsystem
  start at 0.2 s5 : Subsystem
  wires:
  Constant2/1 -> MinMax Running Resettable7/2, MinMax Running Resettable6/2
  Constant1/1 -> MinMax Running Resettable1/2, MinMax Running Resettable5/2
  start at 0.2 s4/1(u) -> MinMax Running Resettable9/1, MinMax Running Resettable8/1
  MinMax Running Resettable7/1 -> Terminator3/1  "Load Voltage Max (pu)"
  Constant3/1 -> MinMax Running Resettable9/2, MinMax Running Resettable8/2
  MinMax Running Resettable8/1 -> Terminator7/1  "Load Current Min (pu)"
  IRMS/1 -> start at 0.2 s4/1(In1)
  MinMax Running Resettable5/1 -> Terminator5/1  "Load Power Max (pu)"
  Active Power/1 -> start at 0.2 s5/1(In1)
  Subsystem4/1(VoltageLow) -> Terminator/1  "Load Voltage Crossed Low"
  start at 0.2 s2/1(u) -> MinMax Running Resettable7/1, MinMax Running Resettable6/1, Subsystem4/1(Voltage)
  Gain/1 -> MinMax Running Resettable5/1, MinMax Running Resettable1/1
  MinMax Running Resettable9/1 -> Terminator6/1  "Load Current Max (pu)"
  start at 0.2 s5/1(u) -> Gain/1
  Subsystem4/2(VoltageHigh) -> Terminator1/1  "Load Voltage Crossed High"
  MinMax Running Resettable6/1 -> Terminator2/1  "Load Voltage Min (pu)"
  MinMax Running Resettable1/1 -> Terminator4/1  "Load Power Min (pu)"
  VRMS/1 -> Low-Pass Filter (Discrete or Continuous)1/1
  Low-Pass Filter (Discrete or Continuous)1/1 -> start at 0.2 s2/1(In1)

== system RemoteMicrogrid/Operator Control Room/Performance and Power Quality/Loss Calculation ==
  Active Power Gen : Inport
  Reactive Power Gen : Inport  Port=2
  Active Power Load : Inport  Port=3
  Reactive Power Load : Inport  Port=4
  Constant4 : Constant  Value=0
  MinMax Running Resettable1 : simulink/Math Operations/MinMax Running Resettable  Function=max  vinit=1
  MinMax Running Resettable2 : simulink/Math Operations/MinMax Running Resettable  Function=max  vinit=1
  Sum : Sum  Inputs=+-
  Sum1 : Sum  Inputs=+-
  Terminator : Terminator
  Terminator1 : Terminator
  start at 2.5 s : Subsystem
  start at 2.5 s1 : Subsystem
  wires:
  start at 2.5 s1/1(u) -> MinMax Running Resettable2/1
  Constant4/1 -> MinMax Running Resettable1/2, MinMax Running Resettable2/2
  Sum/1 -> start at 2.5 s1/1(ActivePower)
  Sum1/1 -> start at 2.5 s/1(ReactivePower)
  MinMax Running Resettable2/1 -> Terminator/1  "Max Active Power Loss (kW)"
  start at 2.5 s/1(u) -> MinMax Running Resettable1/1
  MinMax Running Resettable1/1 -> Terminator1/1  "Max Reactive Power Loss (kW)"
  Active Power Gen/1 -> Sum/1
  Active Power Load/1 -> Sum/2
  Reactive Power Gen/1 -> Sum1/1
  Reactive Power Load/1 -> Sum1/2

== system RemoteMicrogrid/Operator Control Room/Performance and Power Quality/Microgrid Power Quality  ==
  Frequency : Inport
  Voltage : Inport  Port=2
  Constant : Constant  Value=0
  Constant4 : Constant  Value=0
  Low-Pass Filter (Discrete or Continuous) : eeGeneralControl/Low-Pass Filter (Discrete or Continuous)  K=1  T=0.04  B=inf  A=-inf  init_option=Inherited from block input  x0=0  Ts=Ts
  Low-Pass Filter (Discrete or Continuous)1 : eeGeneralControl/Low-Pass Filter (Discrete or Continuous)  K=1  T=0.04  B=inf  A=-inf  init_option=Inherited from block input  x0=0  Ts=Ts
  MinMax Running Resettable : simulink/Math Operations/MinMax Running Resettable  Function=max  vinit=Grid.Frequency
  MinMax Running Resettable2 : simulink/Math Operations/MinMax Running Resettable  Function=max  vinit=1
  MinMax Running Resettable3 : simulink/Math Operations/MinMax Running Resettable  Function=min  vinit=1
  MinMax Running Resettable4 : simulink/Math Operations/MinMax Running Resettable  Function=min  vinit=Grid.Frequency
  Subsystem : Subsystem
  Subsystem3 : Subsystem
  Terminator{,1..7} (8 alike) : Terminator
  start at 2 s : Subsystem
  start at 2 s1 : Subsystem
  wires:
  Subsystem/1(FrequencyLow) -> Terminator/1  "Microgrid Frequency Croosed Low (59 HZ)"
  Constant/1 -> MinMax Running Resettable4/2, MinMax Running Resettable/2
  Frequency/1 -> Low-Pass Filter (Discrete or Continuous)/1
  Subsystem3/1(VoltageLow) -> Terminator4/1  "Microgrid Voltage Crossed Low (0.95 pu)"
  Subsystem/2(FrequencyHigh) -> Terminator1/1  "Microgrid Frequency Crossed High (62 Hz)"
  Voltage/1 -> Low-Pass Filter (Discrete or Continuous)1/1
  MinMax Running Resettable2/1 -> Terminator6/1  "Microgrid Voltage Max (pu)"
  start at 2 s/1(u) -> MinMax Running Resettable4/1, MinMax Running Resettable/1, Subsystem/1(Frequency)
  Subsystem3/2(VoltageHigh) -> Terminator5/1  "Microgrid Voltage Crossed High (1.1 pu)"
  start at 2 s1/1(u) -> MinMax Running Resettable3/1, MinMax Running Resettable2/1, Subsystem3/1(Voltage)
  Constant4/1 -> MinMax Running Resettable3/2, MinMax Running Resettable2/2
  MinMax Running Resettable4/1 -> Terminator3/1  "Microgrid Frequency Min (Hz)"
  MinMax Running Resettable3/1 -> Terminator7/1  "Microgrid Voltage Min (pu)"
  MinMax Running Resettable/1 -> Terminator2/1  "Microgrid Frequency Max (Hz)"
  Low-Pass Filter (Discrete or Continuous)/1 -> start at 2 s/1(In1)
  Low-Pass Filter (Discrete or Continuous)1/1 -> start at 2 s1/1(In1)

== system RemoteMicrogrid/Operator Control Room/Performance and Power Quality/THD ==
  LoadVoltage : Inport
  LoadCurrent : Inport  Port=2
  PCCVoltage : Inport  Port=3
  PCCCurrent : Inport  Port=4
  Terminator{,1..3} (4 alike) : Terminator
  Total Harmonic Distortion{,1..3} (4 alike) : eeTotalHarmonicDistorsion/Total Harmonic Distortion  f=60  Ts=Ts
  wires:
  Total Harmonic Distortion1/1 -> Terminator1/1  "Load Current THD (%)"
  Total Harmonic Distortion3/1 -> Terminator3/1  "PCC Current THD (%)"
  Total Harmonic Distortion2/1 -> Terminator2/1  "PCC Voltage THD (%)"
  Total Harmonic Distortion/1 -> Terminator/1  "Load Voltage THD (%)"
  LoadCurrent/1 -> Total Harmonic Distortion1/1
  LoadVoltage/1 -> Total Harmonic Distortion/1
  PCCVoltage/1 -> Total Harmonic Distortion2/1
  PCCCurrent/1 -> Total Harmonic Distortion3/1

== system RemoteMicrogrid/PV /30 kW PV/L Filter1 ==
  RLC (Three-Phase) : ee_lib/Passive/RLC Assemblies/RLC (Three-Phase)  port_option=ee.enum.threePhasePort.composite  component_structure=ee.enum.rlc.structure.L  R=1e-3 Ohm  L=PV.L H  C=1e-6 F  R_parasitic=0 Ohm  G_parasitic=0 1/Ohm  IL_specify=off  IL_priority=High  IL=[0, 0, 0] A  IL_nominal_specify=off  IL_nominal_value=1  IL_nominal_unit=A  VC_specify=off  VC_priority=High  VC=[0, 0, 0] V  VC_nominal_specify=off  VC_nominal_value=1  VC_nominal_unit=V
      settings: InternalSimscapePortConfiguration="{\"Bottom\":[],\"Left\":[{\"id\":\"N1\",\"label\":\"~1\",\"type\":\"foundation.electrical.three_phase\"}],\"Right\":[{\"id\":\"N2\",\"label\":\"~2\",\"type\":\"foundation.electrical.three_phase\"}],\"Top\":[]}"
  " ~ " : PMIOPort  Side=Right
  ~ : PMIOPort  Port=2  Side=Left
  connections:
  " ~ "/RConn1 -- RLC (Three-Phase)/RConn1
  RLC (Three-Phase)/LConn1 -- ~/RConn1

== system RemoteMicrogrid/PV /30 kW PV/Measurement1 ==
  u : Inport
  Lead-Lag (Discrete or Continuous) : eeGeneralControl/Lead-Lag (Discrete or Continuous)  T1=0  T2=PV.t_sensor  B=inf  A=-inf  init_option=Inherited from block input  x0=0  Ts=Ts
      settings: LibrarySourceBlock=|
      | ee_sl_lib/General Control/Lead-Lag
      | (Discrete or Continuous)
  Out Bus Element : Outport  PortName=ipv1  Element=1
  wires:
  Lead-Lag (Discrete or Continuous)/1 -> Out Bus Element/1
  u/1 -> Lead-Lag (Discrete or Continuous)/1

== system RemoteMicrogrid/PV /30 kW PV/PV Inverter 2 ==
  In Bus Element : Inport  PortName=PV
  In Bus Element1 : Inport  Port=2  PortName=ipv1
  Constant : Constant  Value=1000  SampleTime=-1
  PV Control : Subsystem
  PV Plant : Subsystem
  Conn1 : PMIOPort  Side=Right
  PV power : Outport
  wires:
  Constant/1 -> PV Plant/1(Insolation)
  PV Control/1(mabc) -> PV Plant/2(mod)
  PV Plant/1(PV_plant1) -> PV Control/1(PV_plant1)
  In Bus Element/1 -> PV Control/2(PV)
  In Bus Element1/1 -> PV Control/3(ipv1)
  PV Control/2(PV power) -> PV power/1
  connections:
  Conn1/RConn1 -- PV Plant/RConn1

== system RemoteMicrogrid/PV /PLL & Measurements/Measurement2 ==
  u : Inport
  Lead-Lag (Discrete or Continuous) : eeGeneralControl/Lead-Lag (Discrete or Continuous)  T1=0  T2=PV.t_sensor  B=inf  A=-inf  init_option=Inherited from block input  x0=0  Ts=Ts
      settings: LibrarySourceBlock=|
      | ee_sl_lib/General Control/Lead-Lag
      | (Discrete or Continuous)
  Vg : Outport
  wires:
  Lead-Lag (Discrete or Continuous)/1 -> Vg/1
  u/1 -> Lead-Lag (Discrete or Continuous)/1

== system RemoteMicrogrid/PV /PLL & Measurements/Subsystem ==
  abc : Inport
  Demux : Demux  Outputs=3
  Park Transform : eeTransforms/Park Transform  AxisAlignment=Q-axis  PowerInvariant=off
  "Sinusoidal Measurement (PLL, Three-Phase)1" : eeSinusoidalMeasurementV2/Sinusoidal Measurement (PLL, Three-Phase)  Kp_LF=PV.Kp_pll  Ki_LF=PV.Ki_pll  F0=Grid.Frequency  Theta0=0  Ts=-1
      settings: LibrarySourceBlock=|
      | ee_sl_lib/Measurements/Sinusoidal Measurement
      | (PLL, Three-Phase)
  Terminator : Terminator
  mag : Outport
  freq : Outport  Port=2
  angle : Outport  Port=3
  Vd : Outport  Port=4
  Vq : Outport  Port=5
  wires:
  Demux/3 -> Terminator/1
  abc/1 -> "Sinusoidal Measurement (PLL, Three-Phase)1"/1, Park Transform/1
  Park Transform/1 -> Demux/1
  Demux/1 -> Vd/1
  Demux/2 -> Vq/1
  "Sinusoidal Measurement (PLL, Three-Phase)1"/2 -> Park Transform/2, angle/1
  "Sinusoidal Measurement (PLL, Three-Phase)1"/1 -> freq/1
  "Sinusoidal Measurement (PLL, Three-Phase)1"/3 -> mag/1

== system RemoteMicrogrid/Diesel Substation, BESS, & Microgrid Controller/BESS and Controller/BESS Control/Inverter Active & Reactive Power  ==
  Vabc : Inport
  Iabc : Inport  Port=2
  Demux : Demux  Outputs=3
  Gain : Gain  Gain=1/sqrt(3)
  Minus : Sum  Inputs=+-
  Minus1 : Sum  Inputs=+-
  Minus2 : Sum  Inputs=+-
  Mux : Mux  Inputs=3
  Product : Product
  Product1 : Product
  Sum of Elements : Sum  Inputs=+
  Sum of Elements1 : Sum  Inputs=+
  P : Outport  VectorParamsAs1DForOutWhenUnconnected=off
  Q : Outport  Port=2  VectorParamsAs1DForOutWhenUnconnected=off
  wires:
  Minus/1 -> Mux/3
  Minus2/1 -> Mux/2
  Minus1/1 -> Mux/1
  Sum of Elements1/1 -> Gain/1
  Product1/1 -> Sum of Elements1/1
  Mux/1 -> Product1/2
  Demux/3 -> Minus1/2, Minus2/1
  Demux/2 -> Minus/2, Minus1/1
  Demux/1 -> Minus/1, Minus2/2
  Product/1 -> Sum of Elements/1
  Iabc/1 -> Product/2, Product1/1
  Vabc/1 -> Product/1, Demux/1
  Sum of Elements/1 -> P/1
  Gain/1 -> Q/1

== system RemoteMicrogrid/Diesel Substation, BESS, & Microgrid Controller/Diesel Generator/Governor and Prime Mover /Governor ==
  pu_velocity : Inport
  Load Reference : Inport  Port=2
  1/T_G : Gain  Gain=1/T_G
  1/droop : Gain  Gain=1/(droop_percentage/100)
  Delta load setpoint : Sum  Inputs=+-|
  Delta speed : Sum  Inputs=-+|
  Discrete-Time Integrator1 : DiscreteIntegrator  InitialCondition=pu_torque0  SampleTime=-1  ICPrevOutput=DiscIntNeverNeededParam  ICPrevScaledInput=DiscIntNeverNeededParam
  Speed_ref : Constant  Value=pu_speed_reference
  Subtract : Sum  Inputs=|+-
  delta_y : Outport  VectorParamsAs1DForOutWhenUnconnected=off
  wires:
  Speed_ref/1 -> Delta speed/1
  pu_velocity/1 -> Delta speed/2
  Delta load setpoint/1 -> Subtract/1
  Subtract/1 -> 1/T_G/1
  1/T_G/1 -> Discrete-Time Integrator1/1
  Discrete-Time Integrator1/1 -> delta_y/1, Subtract/2
  Load Reference/1 -> Delta load setpoint/1
  Delta speed/1 -> 1/droop/1
  1/droop/1 -> Delta load setpoint/2

== system RemoteMicrogrid/Diesel Substation, BESS, & Microgrid Controller/Diesel Generator/Governor and Prime Mover /Non-reheat turbine ==
  delta_y : Inport
  1/T_CH : Gain  Gain=1/T_CH
  Discrete-Time Integrator1 : DiscreteIntegrator  InitialCondition=pu_torque0  SampleTime=-1  ICPrevOutput=DiscIntNeverNeededParam  ICPrevScaledInput=DiscIntNeverNeededParam
  Sum : Sum  Inputs=|+-
  torque : Outport  VectorParamsAs1DForOutWhenUnconnected=off
  wires:
  delta_y/1 -> Sum/1
  Sum/1 -> 1/T_CH/1
  1/T_CH/1 -> Discrete-Time Integrator1/1
  Discrete-Time Integrator1/1 -> Sum/2, torque/1

== system RemoteMicrogrid/Diesel Substation, BESS, & Microgrid Controller/Microgrid Controller/Microgrid Supervisory Control/Transition and Dispatch Control/On.Planned_Islanding ==
  PlannedIslanding : Inport
  " Demux " : Demux  Outputs=1
  " SFunction " : S-Function  Tag=Stateflow S-Function 1  FunctionName=sf_sfun  PortCounts=[1 5]  SFunctionDeploymentMode=off  EnableBusSupport=off
  " Terminator " : Terminator
  PCC : Outport
  plannedIslanding : Outport  Port=2
  plannedIslandingDispatch : Outport  Port=3
  plannedIslandingStatus : Outport  Port=4
  wires:
  PlannedIslanding/1 -> " SFunction "/1
  " SFunction "/2 -> PCC/1  "PCC"
  " SFunction "/3 -> plannedIslanding/1  "plannedIslanding"
  " SFunction "/4 -> plannedIslandingDispatch/1  "plannedIslandingDispatch"
  " SFunction "/5 -> plannedIslandingStatus/1  "plannedIslandingStatus"
  " Demux "/1 -> " Terminator "/1
  " SFunction "/1 -> " Demux "/1

== system RemoteMicrogrid/Diesel Substation, BESS, & Microgrid Controller/Microgrid Controller/Microgrid Supervisory Control/Transition and Dispatch Control/On.Resynchronization ==
  Resync : Inport
  " Demux " : Demux  Outputs=1
  " SFunction " : S-Function  Tag=Stateflow S-Function 7  FunctionName=sf_sfun  PortCounts=[1 5]  SFunctionDeploymentMode=off  EnableBusSupport=off
  " Terminator " : Terminator
  PCC : Outport
  resync : Outport  Port=2
  resyncDispatch : Outport  Port=3
  resyncStatus : Outport  Port=4
  wires:
  Resync/1 -> " SFunction "/1
  " SFunction "/2 -> PCC/1  "PCC"
  " SFunction "/3 -> resync/1  "resync"
  " SFunction "/4 -> resyncDispatch/1  "resyncDispatch"
  " SFunction "/5 -> resyncStatus/1  "resyncStatus"
  " Demux "/1 -> " Terminator "/1
  " SFunction "/1 -> " Demux "/1

== system RemoteMicrogrid/Diesel Substation, BESS, & Microgrid Controller/Microgrid Controller/Microgrid Supervisory Control/Transition and Dispatch Control/On.Steady_State_Grid_Connected ==
  resyncDispatch : Inport
  " Demux " : Demux  Outputs=1
  " SFunction " : S-Function  Tag=Stateflow S-Function 5  FunctionName=sf_sfun  PortCounts=[1 6]  SFunctionDeploymentMode=off  EnableBusSupport=off
  " Terminator " : Terminator
  LoadF2A : Outport
  LoadF2B : Outport  Port=2
  loadDispatch : Outport  Port=3
  loadReference : Outport  Port=4
  emergencyDispatch : Outport  Port=5
  wires:
  resyncDispatch/1 -> " SFunction "/1
  " SFunction "/2 -> LoadF2A/1  "LoadF2A"
  " SFunction "/3 -> LoadF2B/1  "LoadF2B"
  " SFunction "/4 -> loadDispatch/1  "loadDispatch"
  " SFunction "/5 -> loadReference/1  "loadReference"
  " SFunction "/6 -> emergencyDispatch/1  "emergencyDispatch"
  " Demux "/1 -> " Terminator "/1
  " SFunction "/1 -> " Demux "/1

== system RemoteMicrogrid/Diesel Substation, BESS, & Microgrid Controller/Microgrid Controller/Microgrid Supervisory Control/Transition and Dispatch Control/On.Steady_State_Islanded ==
  plannedIslandingDispatch : Inport
  " Demux " : Demux  Outputs=1
  " SFunction " : S-Function  Tag=Stateflow S-Function 8  FunctionName=sf_sfun  PortCounts=[1 5]  SFunctionDeploymentMode=off  EnableBusSupport=off
  " Terminator " : Terminator
  LoadF2A : Outport
  LoadF2B : Outport  Port=2
  loadDispatch : Outport  Port=3
  emergencyDispatch : Outport  Port=4
  wires:
  plannedIslandingDispatch/1 -> " SFunction "/1
  " SFunction "/2 -> LoadF2A/1  "LoadF2A"
  " SFunction "/3 -> LoadF2B/1  "LoadF2B"
  " SFunction "/4 -> loadDispatch/1  "loadDispatch"
  " SFunction "/5 -> emergencyDispatch/1  "emergencyDispatch"
  " Demux "/1 -> " Terminator "/1
  " SFunction "/1 -> " Demux "/1
